simulink library "TripedLibrary"  (R2021a)
settings: Solver=VariableStepAuto  StartTime=0.0  StopTime=10.0  RelTol=1e-3
values from neighbouring files (symbols this model uses):
  s = 1/(2*r)    [Weg0.m]
undefined symbols (not defined in the file or in its folder): X, Y, Z
libraries: sm_lib x95, nesl_utility x42, $bdroot x14, robotlib x9, simulink x6, spsFirstOrderFilterLib x3, mspsensorlib x1
(part 5 of 5)

== matlab function TripedLibrary/Kinematic Utils/Simplified  Model Kinematics/Fwd Kin ==
  data: Jointstate input; leg_pos output; LegNumber input
function leg_pos = fcn(Jointstate, LegNumber)
waym = Weg0(eul2quat(Jointstate(1:3).','XYZ'));
wayLLm = AddLegLinear(waym,Jointstate(4));
legstate = getPosfromHomogenMatrix(wayLLm);
leg_pos = transformCoordinateSystem(legstate(1),legstate(2),legstate(3),LegNumber);
end




function [new_pos] = transformCoordinateSystem(oldx,oldy,oldz,legNr)
% this function translates the x,y,z coordinates from the CCS into
% coordinates from a cooridnate system, which is like the ccs but rotated
% ,such that its x axis points towards the leg. This makes the inverse
% kinematics for the leg 1 & 2 easier.

angle = -legNr * 120 * pi/180;

newCoord = [cos(angle), -sin(angle), 0, 0; sin(angle), cos(angle), 0, 0; 0, 0, 1, 0; 0, 0, 0, 1]* [oldx;oldy;oldz;1];
newx = newCoord(1);
newy = newCoord(2);
newz = newCoord(3);

new_pos=[newx;newy;newz];
end

function [Weg0Mat] = Weg0(quat)
a0=quat(1);
b0=quat(2);
c0=quat(3);
d0=quat(4);
A1 = homogenTranslationMat(0.265,0,0.014);
A2 = makeRotHomogen(quatRotM(a0,b0,c0,d0));
Weg0Mat = A1 * A2;
end



function [ALeg] = AddLegLinear(A,theta0)
% this functions adds transformations from the Point P; which is the
% Endpoint from Weg0,1,2; to the FKS at the LegLinear part.
%{
Inputs:
A: Transformationmatrix, which describes Transformation from HKS to P, Use
Weg0.m for that.
theta0: angle [radians] for joint at MKS00
%}

A1 = homogenTranslationMat(1.640, 0, -0.037); % transform P to P0 (center of LegLinear rotation)

theta0 = -1* theta0 * 0.07/(2*pi*1.5); % gear constraint: transfrom theta at MKS00 to theta around P0, gear ratio is 0.07/(2*pi*1.5) [circumferences of the gears MCS00 / LL]
startingvalue = -0 * pi/180;
theta0 = theta0 + startingvalue; %offset, depending on which position the Leg is for theta at MKS00 is 0
A2 = makeRotHomogen(quatRotM(cos(theta0/2),0,sin(theta0/2),0)); % rotate theta [radians] around y-axis of P0

A3 = homogenTranslationMat(-1.500,0,0); %transform from P0-joint to FKS

ALeg = A*A1*A2*A3;
end

function [res] = homogenTranslationMat(x,y,z)
    %this function forms a Translation about a vector x,y,z in a homogenous
    %transformation matrix res. 
    res = [1 0 0 x; 0 1 0 y; 0 0 1 z; 0 0 0 1];
end

function [res] = makeRotHomogen(R)
% this function fills a Rotationmatrix to make it a homogen transformation
% matrix
res = [R(1,1) R(1,2) R(1,3) 0; R(2,1) R(2,2) R(2,3) 0; R(3,1) R(3,2) R(3,3) 0; 0 0 0 1];
end

function [res] = quatRotM(a,b,c,d) %%Todo: use a,b,c,d as inputs
    % this function calculates the quaternion rotation matrix for given
    % vector (kx,ky,kz) and angle theta
    res = [1-2*(c^2+d^2) 2*(b*c-d*a) 2*(b*d + c*a); 2*(b*c + d*a) 1-2*(b^2+d^2) 2*(c*d - b*a); 2*(b*d-c*a) 2*(c*d+b*a) 1-2*(b^2+c^2) ];
end




function [pos] = getPosfromHomogenMatrix(A)
    % this function returns the Vector by which a homogenous
    % Transformationmatrix shifts a Point
    x = A(1,4);
    y = A(2,4);
    z = A(3,4);

    pos=[x,y,z];
end

== matlab function TripedLibrary/Kinematic Utils/Simplified  Model Kinematics/Inv Kin/Simplified_inverse_kinematics ==
  data: extend output; Rx output; Ry output; x input; y input; z input; LegAngle input; Rz output; data input; Residual output
function [extend,Rx,Ry,Rz,Residual]= fcn(x,y,z,LegAngle, data)



% easy adapt to legs 1 & 2: change base coordinate system from ccs, to
% rotated ccs.
[newx,newy,newz] = transformCoordinateSystem(x,y,z,LegAngle);

% calculate target Matrix from input cordinates
%reduced task space to x,y,z, ignore roll, pitch, yaw
[targetM] = convertCoordinatesToMatrix(newx,newy,newz);

%convert euer angles from data to quaternion
guess = convertDataToGuess(data);

[extend, a0,b0,c0,d0, Residual] = inverseKinematics(targetM,guess);
eulerXYZ = quat2eul([a0,b0,c0,d0],'XYZ');
Rx = eulerXYZ(1);
Ry = eulerXYZ(2);
Rz = eulerXYZ(3);

end

function [newx,newy,newz] = transformCoordinateSystem(oldx,oldy,oldz,legAngle)
% this function translates the x,y,z coordinates from the CCS into
% coordinates from a cooridnate system, which is like the ccs but rotated
% ,such that its x axis points towards the leg. This makes the inverse
% kinematics for the leg 1 & 2 easier.

angle = legAngle;

newCoord = [cos(angle), -sin(angle), 0, 0; sin(angle), cos(angle), 0, 0; 0, 0, 1, 0; 0, 0, 0, 1]* [oldx;oldy;oldz;1];
newx = newCoord(1);
newy = newCoord(2);
newz = newCoord(3);

end

function [transfM] = convertCoordinatesToMatrix(x,y,z)
transfM = homogenTranslationMat(x,y,z);
end

function [guess] = convertDataToGuess(data)
    qXYZ = eul2quat([data(1),data(2),data(3)],'XYZ');
    guess = [qXYZ,data(4)];    
end

function [theta0,a0,b0,c0,d0,fvalWay0] = inverseKinematics(A,guess)
% maps a homogene transformation matrix, which describes the desired position
% of the fcs relative to the ccs in taskspace to the joint space variables


options = optimoptions(@fmincon,'OptimalityTolerance',10^-10,'StepTolerance',10^-10,'display','off','Algorithm','sqp'); % some options for more precise solution


guessVals = guess;

clW0toTarget = @(guessVals)closingWay0toTarget(guessVals,A);
[OptVals,fvalWay0,~,~] = fmincon(clW0toTarget,guessVals,[],[],[],[],[],[],@constrainsWay0,options);

% get values from way0
a0 = OptVals(1);
b0 = OptVals(2);
c0 = OptVals(3);
d0 = OptVals(4);
theta0 = OptVals(5);

end


function [error] = closingWay0toTarget(GUESSEDVALS,MatA)
% this function returns the error between the desired fcs position and the
% fcs position given GUESSEDVALS as joint values

a0 = GUESSEDVALS(1);
b0 = GUESSEDVALS(2);
c0 = GUESSEDVALS(3);
d0 = GUESSEDVALS(4);
theta0 = GUESSEDVALS(5);

way0m = Weg0(a0,b0,c0,d0);
way0LLm = AddLegLinear(way0m,theta0);
[a,b,c,d, x,y,z] = getValuesfromHomogenMatrix(way0LLm);
[~,~,~,~, Ax,Ay,Az] = getValuesfromHomogenMatrix(MatA);


% give the system a desired yaw of the leg, since it is highly redundant
% this makes the solution more predictable

[~,desired_orientation]= cart2pol(Ax-0.265,Ay);
current_orientation = quat2eul([a0,b0,c0,d0]);


error = sum(([x,y,z] - [Ax,Ay,Az]).^2) + 1*(a^2+b^2+c^2+d^2 -1)^2+10*(desired_orientation-current_orientation(1))^2; % error of the transform to A. we want to minimze this
end


function [c,ceq]= constrainsWay0(x)
% make sure that solver fmincon considers that the quaternion a0,b0,c0,d0
% needs to be normalized.
%input: x = [a0,b0,c0,d0,theta0].
c = []; % condition for ... <= 0
ceq = x(1)^2+x(2)^2+x(3)^2+x(4)^2 - 1; % condition for ||quat0|| == 1    
end

function [Weg0Mat] = Weg0(a0,b0,c0,d0)
A1 = homogenTranslationMat(0.265,0,0.014);
A2 = makeRotHomogen(quatRotM(a0,b0,c0,d0));
Weg0Mat = A1 * A2;
end

function [ALeg] = AddLegLinear(A,theta0)
% this functions adds transformations from the Point P; which is the
% Endpoint from Weg0,1,2; to the FKS at the LegLinear part.
%{
Inputs:
A: Transformationmatrix, which describes Transformation from HKS to P, Use
Weg0.m for that.
theta0: angle [radians] for joint at MKS00
%}

A1 = homogenTranslationMat(1.640, 0, -0.037); 

theta0 = -1* theta0 * 0.07/(2*pi*1.5); % gear constraint between motor and curved leg
startingvalue = -0 * pi/180;
theta0 = theta0 + startingvalue;
A2 = makeRotHomogen(quatRotM(cos(theta0/2),0,sin(theta0/2),0)); 
A3 = homogenTranslationMat(-1.500,0,0);

ALeg = A*A1*A2*A3;
end

function [res] = homogenTranslationMat(x,y,z)
    %this function forms a Translation about a vector x,y,z in a homogenous
    %transformation matrix res. 
    res = [1 0 0 x; 0 1 0 y; 0 0 1 z; 0 0 0 1];
end

function [res] = makeRotHomogen(R)
% this function fills a Rotationmatrix to make it a homogen transformation
% matrix
res = [R(1,1) R(1,2) R(1,3) 0; R(2,1) R(2,2) R(2,3) 0; R(3,1) R(3,2) R(3,3) 0; 0 0 0 1];
end

function [res] = quatRotM(a,b,c,d) %%Todo: use a,b,c,d as inputs
    res = [1-2*(c^2+d^2) 2*(b*c-d*a) 2*(b*d + c*a); 2*(b*c + d*a) 1-2*(b^2+d^2) 2*(c*d - b*a); 2*(b*d-c*a) 2*(c*d+b*a) 1-2*(b^2+c^2) ];
end

function [a,b,c,d, x,y,z] = getValuesfromHomogenMatrix(A)
    % this function returns the Vector by which a homogenous
    % Transformationmatrix shifts a Point
    x = A(1,4);
    y = A(2,4);
    z = A(3,4);

    %as well as the Values of the Quaternion describing the rotation
    R = A(1:3,1:3); % get Rot mat from homogen Mat
    quat = rotm2quat(R);
    a = quat(1);
    b = quat(2);
    c = quat(3);
    d = quat(4); 
end

== matlab function TripedLibrary/Kinematic Utils/fullbody kinematics ==
  data: foot0 input; res output; foot1 input; foot2 input; roll input; pitch input; yaw input; height input
function res  = fcn(foot0,foot1,foot2,roll,pitch,yaw,height)
floor_ccs_trafo=transform_to_floor(roll,pitch,yaw,height);

ccs_foot0=floor_ccs_trafo*makehomogenous(foot0);
ccs_foot1=floor_ccs_trafo*makehomogenous(foot1);
ccs_foot2=floor_ccs_trafo*makehomogenous(foot2);
res=[ccs_foot0(1:3);ccs_foot1(1:3);ccs_foot2(1:3)];
end


function [transfM] = transform_to_floor(roll,pitch,yaw,height)
%first translate frame by [x,y,z]
transfM1 = homogenTranslationMat(0,0,-height);
%then rotate using the roll-pitch-yaw convention
transfM2 = makeRotHomogen(eul2rotm([-roll,-pitch,-yaw],'XYZ'));
transfM = transfM1 * transfM2;
end

function [res] = makehomogenous(vector)
    res = [vector(1);vector(2);vector(3);1];
end

function [res] = homogenTranslationMat(x,y,z)
    %this function forms a Translation about a vector x,y,z in a homogenous
    %transformation matrix res. 
    res = [1 0 0 x; 0 1 0 y; 0 0 1 z; 0 0 0 1];
end

function [res] = makeRotHomogen(R)
% this function fills a Rotationmatrix to make it a homogen transformation
% matrix
res = [R(1,1) R(1,2) R(1,3) 0; R(2,1) R(2,2) R(2,3) 0; R(3,1) R(3,2) R(3,3) 0; 0 0 0 1];
end

== matlab function TripedLibrary/Simplified Model/TriPed/Forward Kinematics/MATLAB Function ==
  data: Jointstate input; leg_pos output; LegNumber input
function leg_pos = fcn(Jointstate, LegNumber)
waym = Weg0(eul2quat(Jointstate(1:3).','XYZ'));
wayLLm = AddLegLinear(waym,Jointstate(4));
legstate = getPosfromHomogenMatrix(wayLLm);
leg_pos = transformCoordinateSystem(legstate(1),legstate(2),legstate(3),LegNumber);
end




function [new_pos] = transformCoordinateSystem(oldx,oldy,oldz,legNr)
% this function translates the x,y,z coordinates from the CCS into
% coordinates from a cooridnate system, which is like the ccs but rotated
% ,such that its x axis points towards the leg. This makes the inverse
% kinematics for the leg 1 & 2 easier.

angle = -legNr * 120 * pi/180;

newCoord = [cos(angle), -sin(angle), 0, 0; sin(angle), cos(angle), 0, 0; 0, 0, 1, 0; 0, 0, 0, 1]* [oldx;oldy;oldz;1];
newx = newCoord(1);
newy = newCoord(2);
newz = newCoord(3);

new_pos=[newx;newy;newz];
end

function [Weg0Mat] = Weg0(quat)
a0=quat(1);
b0=quat(2);
c0=quat(3);
d0=quat(4);
A1 = homogenTranslationMat(0.265,0,0.014);
A2 = makeRotHomogen(quatRotM(a0,b0,c0,d0));
Weg0Mat = A1 * A2;
end



function [ALeg] = AddLegLinear(A,theta0)
% this functions adds transformations from the Point P; which is the
% Endpoint from Weg0,1,2; to the FKS at the LegLinear part.
%{
Inputs:
A: Transformationmatrix, which describes Transformation from HKS to P, Use
Weg0.m for that.
theta0: angle [radians] for joint at MKS00
%}

A1 = homogenTranslationMat(1.640, 0, -0.037); % transform P to P0 (center of LegLinear rotation)

theta0 = -1* theta0 * 0.07/(2*pi*1.5); % gear constraint: transfrom theta at MKS00 to theta around P0, gear ratio is 0.07/(2*pi*1.5) [circumferences of the gears MCS00 / LL]
startingvalue = -0 * pi/180;
theta0 = theta0 + startingvalue; %offset, depending on which position the Leg is for theta at MKS00 is 0
A2 = makeRotHomogen(quatRotM(cos(theta0/2),0,sin(theta0/2),0)); % rotate theta [radians] around y-axis of P0

A3 = homogenTranslationMat(-1.500,0,0); %transform from P0-joint to FKS

ALeg = A*A1*A2*A3;
end

function [res] = homogenTranslationMat(x,y,z)
    %this function forms a Translation about a vector x,y,z in a homogenous
    %transformation matrix res. 
    res = [1 0 0 x; 0 1 0 y; 0 0 1 z; 0 0 0 1];
end

function [res] = makeRotHomogen(R)
% this function fills a Rotationmatrix to make it a homogen transformation
% matrix
res = [R(1,1) R(1,2) R(1,3) 0; R(2,1) R(2,2) R(2,3) 0; R(3,1) R(3,2) R(3,3) 0; 0 0 0 1];
end

function [res] = quatRotM(a,b,c,d) %%Todo: use a,b,c,d as inputs
    % this function calculates the quaternion rotation matrix for given
    % vector (kx,ky,kz) and angle theta
    res = [1-2*(c^2+d^2) 2*(b*c-d*a) 2*(b*d + c*a); 2*(b*c + d*a) 1-2*(b^2+d^2) 2*(c*d - b*a); 2*(b*d-c*a) 2*(c*d+b*a) 1-2*(b^2+c^2) ];
end




function [pos] = getPosfromHomogenMatrix(A)
    % this function returns the Vector by which a homogenous
    % Transformationmatrix shifts a Point
    x = A(1,4);
    y = A(2,4);
    z = A(3,4);

    pos=[x,y,z];
end

== matlab function TripedLibrary/Full Model/ROS/Publisher_leg_0/Sensor_Publisher/mergeValuesIntoRosMsg_test ==
  data: blankMessage input Bus: SL_Bus_triped_sensor_msgs_JointState; position input; msg output Bus: SL_Bus_triped_sensor_msgs_JointState
function msg = assignNestedArrayMessages(blankMessage,position)
%#codegen

% To set datatype of MSG output:
%  1. Create buses for this model: robotics.ros.createSimulinkBus(gcs)
%  1. Click "Edit Data" in  Toolstrip to open "Ports and Data Manager"
%  2. Select MSG and set datatype to "Bus: SL_Bus_<modelname>_<messageType>"
% See: 
% http://www.mathworks.com/help/simulink/ug/create-structures-in-matlab-function-blocks.html

% blankMessage (geometry_msgs/PoseArray) consists of
%          Header: [1x1 Header]
%           Poses: variable-length array of geometry_msgs/Pose
%   Poses_SL_Info: struct with fields CurrentLength, ReceivedLength
%
% Poses is an array of "geometry_msgs/Pose", which consists of
%        Position: [1x1 Point]
%     Orientation: [1x1 Quaternion]
%
% Position is "geometry_msgs/Point", which consists of
%               X: 0
%               Y: 0
%               Z: 0
%
% Orientation is "geometry_msgs/Quaternion", which consists of
%               X: 0
%               Y: 0
%               Z: 0
%               W: 0

% Set the Poses array to have size 2, and modify the first two Pose
% elements

%blankMessage.Poses_SL_Info.CurrentLength = uint32(2);
%blankMessage.Poses(1).Position.X = x;
%blankMessage.Poses(1).Position.Y = y;
%blankMessage.Poses(2).Orientation.Z = z;

blankMessage.Position_SL_Info.CurrentLength = uint32(1);
%blankMessage.Velocity_SL_Info.CurrentLength = uint32(2);
%blankMessage.Effort_SL_Info.CurrentLength = uint32(2);
blankMessage.Position(1) = position;
%blankMessage.Velocity(2) = velocity;
%blankMessage.Position(2) = effort;

msg = blankMessage;

== matlab function TripedLibrary/Simplified Model/TriPed/Forward Kinematics/MATLAB Function1 ==
  data: Jointstate input; leg_pos output; LegNumber input
function leg_pos = fcn(Jointstate, LegNumber)
waym = Weg0(eul2quat(Jointstate(1:3).','XYZ'));
wayLLm = AddLegLinear(waym,Jointstate(4));
legstate = getPosfromHomogenMatrix(wayLLm);
leg_pos = transformCoordinateSystem(legstate(1),legstate(2),legstate(3),LegNumber);
end




function [new_pos] = transformCoordinateSystem(oldx,oldy,oldz,legNr)
% this function translates the x,y,z coordinates from the CCS into
% coordinates from a cooridnate system, which is like the ccs but rotated
% ,such that its x axis points towards the leg. This makes the inverse
% kinematics for the leg 1 & 2 easier.

angle = -legNr * 120 * pi/180;

newCoord = [cos(angle), -sin(angle), 0, 0; sin(angle), cos(angle), 0, 0; 0, 0, 1, 0; 0, 0, 0, 1]* [oldx;oldy;oldz;1];
newx = newCoord(1);
newy = newCoord(2);
newz = newCoord(3);

new_pos=[newx;newy;newz];
end

function [Weg0Mat] = Weg0(quat)
a0=quat(1);
b0=quat(2);
c0=quat(3);
d0=quat(4);
A1 = homogenTranslationMat(0.265,0,0.014);
A2 = makeRotHomogen(quatRotM(a0,b0,c0,d0));
Weg0Mat = A1 * A2;
end



function [ALeg] = AddLegLinear(A,theta0)
% this functions adds transformations from the Point P; which is the
% Endpoint from Weg0,1,2; to the FKS at the LegLinear part.
%{
Inputs:
A: Transformationmatrix, which describes Transformation from HKS to P, Use
Weg0.m for that.
theta0: angle [radians] for joint at MKS00
%}

A1 = homogenTranslationMat(1.640, 0, -0.037); % transform P to P0 (center of LegLinear rotation)

theta0 = -1* theta0 * 0.07/(2*pi*1.5); % gear constraint: transfrom theta at MKS00 to theta around P0, gear ratio is 0.07/(2*pi*1.5) [circumferences of the gears MCS00 / LL]
startingvalue = -0 * pi/180;
theta0 = theta0 + startingvalue; %offset, depending on which position the Leg is for theta at MKS00 is 0
A2 = makeRotHomogen(quatRotM(cos(theta0/2),0,sin(theta0/2),0)); % rotate theta [radians] around y-axis of P0

A3 = homogenTranslationMat(-1.500,0,0); %transform from P0-joint to FKS

ALeg = A*A1*A2*A3;
end

function [res] = homogenTranslationMat(x,y,z)
    %this function forms a Translation about a vector x,y,z in a homogenous
    %transformation matrix res. 
    res = [1 0 0 x; 0 1 0 y; 0 0 1 z; 0 0 0 1];
end

function [res] = makeRotHomogen(R)
% this function fills a Rotationmatrix to make it a homogen transformation
% matrix
res = [R(1,1) R(1,2) R(1,3) 0; R(2,1) R(2,2) R(2,3) 0; R(3,1) R(3,2) R(3,3) 0; 0 0 0 1];
end

function [res] = quatRotM(a,b,c,d) %%Todo: use a,b,c,d as inputs
    % this function calculates the quaternion rotation matrix for given
    % vector (kx,ky,kz) and angle theta
    res = [1-2*(c^2+d^2) 2*(b*c-d*a) 2*(b*d + c*a); 2*(b*c + d*a) 1-2*(b^2+d^2) 2*(c*d - b*a); 2*(b*d-c*a) 2*(c*d+b*a) 1-2*(b^2+c^2) ];
end




function [pos] = getPosfromHomogenMatrix(A)
    % this function returns the Vector by which a homogenous
    % Transformationmatrix shifts a Point
    x = A(1,4);
    y = A(2,4);
    z = A(3,4);

    pos=[x,y,z];
end

== matlab function TripedLibrary/Simplified Model/TriPed/Forward Kinematics/MATLAB Function2 ==
  data: Jointstate input; leg_pos output; LegNumber input
function leg_pos = fcn(Jointstate, LegNumber)
waym = Weg0(eul2quat(Jointstate(1:3).','XYZ'));
wayLLm = AddLegLinear(waym,Jointstate(4));
legstate = getPosfromHomogenMatrix(wayLLm);
leg_pos = transformCoordinateSystem(legstate(1),legstate(2),legstate(3),LegNumber);
end




function [new_pos] = transformCoordinateSystem(oldx,oldy,oldz,legNr)
% this function translates the x,y,z coordinates from the CCS into
% coordinates from a cooridnate system, which is like the ccs but rotated
% ,such that its x axis points towards the leg. This makes the inverse
% kinematics for the leg 1 & 2 easier.

angle = -legNr * 120 * pi/180;

newCoord = [cos(angle), -sin(angle), 0, 0; sin(angle), cos(angle), 0, 0; 0, 0, 1, 0; 0, 0, 0, 1]* [oldx;oldy;oldz;1];
newx = newCoord(1);
newy = newCoord(2);
newz = newCoord(3);

new_pos=[newx;newy;newz];
end

function [Weg0Mat] = Weg0(quat)
a0=quat(1);
b0=quat(2);
c0=quat(3);
d0=quat(4);
A1 = homogenTranslationMat(0.265,0,0.014);
A2 = makeRotHomogen(quatRotM(a0,b0,c0,d0));
Weg0Mat = A1 * A2;
end



function [ALeg] = AddLegLinear(A,theta0)
% this functions adds transformations from the Point P; which is the
% Endpoint from Weg0,1,2; to the FKS at the LegLinear part.
%{
Inputs:
A: Transformationmatrix, which describes Transformation from HKS to P, Use
Weg0.m for that.
theta0: angle [radians] for joint at MKS00
%}

A1 = homogenTranslationMat(1.640, 0, -0.037); % transform P to P0 (center of LegLinear rotation)

theta0 = -1* theta0 * 0.07/(2*pi*1.5); % gear constraint: transfrom theta at MKS00 to theta around P0, gear ratio is 0.07/(2*pi*1.5) [circumferences of the gears MCS00 / LL]
startingvalue = -0 * pi/180;
theta0 = theta0 + startingvalue; %offset, depending on which position the Leg is for theta at MKS00 is 0
A2 = makeRotHomogen(quatRotM(cos(theta0/2),0,sin(theta0/2),0)); % rotate theta [radians] around y-axis of P0

A3 = homogenTranslationMat(-1.500,0,0); %transform from P0-joint to FKS

ALeg = A*A1*A2*A3;
end

function [res] = homogenTranslationMat(x,y,z)
    %this function forms a Translation about a vector x,y,z in a homogenous
    %transformation matrix res. 
    res = [1 0 0 x; 0 1 0 y; 0 0 1 z; 0 0 0 1];
end

function [res] = makeRotHomogen(R)
% this function fills a Rotationmatrix to make it a homogen transformation
% matrix
res = [R(1,1) R(1,2) R(1,3) 0; R(2,1) R(2,2) R(2,3) 0; R(3,1) R(3,2) R(3,3) 0; 0 0 0 1];
end

function [res] = quatRotM(a,b,c,d) %%Todo: use a,b,c,d as inputs
    % this function calculates the quaternion rotation matrix for given
    % vector (kx,ky,kz) and angle theta
    res = [1-2*(c^2+d^2) 2*(b*c-d*a) 2*(b*d + c*a); 2*(b*c + d*a) 1-2*(b^2+d^2) 2*(c*d - b*a); 2*(b*d-c*a) 2*(c*d+b*a) 1-2*(b^2+c^2) ];
end




function [pos] = getPosfromHomogenMatrix(A)
    % this function returns the Vector by which a homogenous
    % Transformationmatrix shifts a Point
    x = A(1,4);
    y = A(2,4);
    z = A(3,4);

    pos=[x,y,z];
end

== matlab function TripedLibrary/Full Model/ROS/Publisher_leg_0/Sensor_Publisher1/mergeValuesIntoRosMsg_test ==
  data: blankMessage input Bus: SL_Bus_triped_sensor_msgs_JointState; position input; msg output Bus: SL_Bus_triped_sensor_msgs_JointState
function msg = assignNestedArrayMessages(blankMessage,position)
%#codegen

% To set datatype of MSG output:
%  1. Create buses for this model: robotics.ros.createSimulinkBus(gcs)
%  1. Click "Edit Data" in  Toolstrip to open "Ports and Data Manager"
%  2. Select MSG and set datatype to "Bus: SL_Bus_<modelname>_<messageType>"
% See: 
% http://www.mathworks.com/help/simulink/ug/create-structures-in-matlab-function-blocks.html

% blankMessage (geometry_msgs/PoseArray) consists of
%          Header: [1x1 Header]
%           Poses: variable-length array of geometry_msgs/Pose
%   Poses_SL_Info: struct with fields CurrentLength, ReceivedLength
%
% Poses is an array of "geometry_msgs/Pose", which consists of
%        Position: [1x1 Point]
%     Orientation: [1x1 Quaternion]
%
% Position is "geometry_msgs/Point", which consists of
%               X: 0
%               Y: 0
%               Z: 0
%
% Orientation is "geometry_msgs/Quaternion", which consists of
%               X: 0
%               Y: 0
%               Z: 0
%               W: 0

% Set the Poses array to have size 2, and modify the first two Pose
% elements

%blankMessage.Poses_SL_Info.CurrentLength = uint32(2);
%blankMessage.Poses(1).Position.X = x;
%blankMessage.Poses(1).Position.Y = y;
%blankMessage.Poses(2).Orientation.Z = z;

blankMessage.Position_SL_Info.CurrentLength = uint32(1);
%blankMessage.Velocity_SL_Info.CurrentLength = uint32(2);
%blankMessage.Effort_SL_Info.CurrentLength = uint32(2);
blankMessage.Position(1) = position;
%blankMessage.Velocity(2) = velocity;
%blankMessage.Position(2) = effort;

msg = blankMessage;

== matlab function TripedLibrary/Full Model/ROS/Publisher_leg_0/Sensor_Publisher2/mergeValuesIntoRosMsg_test ==
  data: blankMessage input Bus: SL_Bus_triped_sensor_msgs_JointState; position input; msg output Bus: SL_Bus_triped_sensor_msgs_JointState
function msg = assignNestedArrayMessages(blankMessage,position)
%#codegen

% To set datatype of MSG output:
%  1. Create buses for this model: robotics.ros.createSimulinkBus(gcs)
%  1. Click "Edit Data" in  Toolstrip to open "Ports and Data Manager"
%  2. Select MSG and set datatype to "Bus: SL_Bus_<modelname>_<messageType>"
% See: 
% http://www.mathworks.com/help/simulink/ug/create-structures-in-matlab-function-blocks.html

% blankMessage (geometry_msgs/PoseArray) consists of
%          Header: [1x1 Header]
%           Poses: variable-length array of geometry_msgs/Pose
%   Poses_SL_Info: struct with fields CurrentLength, ReceivedLength
%
% Poses is an array of "geometry_msgs/Pose", which consists of
%        Position: [1x1 Point]
%     Orientation: [1x1 Quaternion]
%
% Position is "geometry_msgs/Point", which consists of
%               X: 0
%               Y: 0
%               Z: 0
%
% Orientation is "geometry_msgs/Quaternion", which consists of
%               X: 0
%               Y: 0
%               Z: 0
%               W: 0

% Set the Poses array to have size 2, and modify the first two Pose
% elements

%blankMessage.Poses_SL_Info.CurrentLength = uint32(2);
%blankMessage.Poses(1).Position.X = x;
%blankMessage.Poses(1).Position.Y = y;
%blankMessage.Poses(2).Orientation.Z = z;

blankMessage.Position_SL_Info.CurrentLength = uint32(1);
%blankMessage.Velocity_SL_Info.CurrentLength = uint32(2);
%blankMessage.Effort_SL_Info.CurrentLength = uint32(2);
blankMessage.Position(1) = position;
%blankMessage.Velocity(2) = velocity;
%blankMessage.Position(2) = effort;

msg = blankMessage;

== matlab function TripedLibrary/Examples/Full Body orientation and height control/fullbody kinematics ==
  data: foot0 input; res output; foot1 input; foot2 input; roll input; pitch input; yaw input; height input
function res  = fcn(foot0,foot1,foot2,roll,pitch,yaw,height)
floor_ccs_trafo=transform_to_floor(roll,pitch,yaw,height);

ccs_foot0=floor_ccs_trafo*makehomogenous(foot0);
ccs_foot1=floor_ccs_trafo*makehomogenous(foot1);
ccs_foot2=floor_ccs_trafo*makehomogenous(foot2);
res=[ccs_foot0(1:3);ccs_foot1(1:3);ccs_foot2(1:3)];
end


function [transfM] = transform_to_floor(roll,pitch,yaw,height)
%first translate frame by [x,y,z]
transfM1 = homogenTranslationMat(0,0,-height);
%then rotate using the roll-pitch-yaw convention
transfM2 = makeRotHomogen(eul2rotm([-roll,-pitch,-yaw],'XYZ'));
transfM = transfM1 * transfM2;
end

function [res] = makehomogenous(vector)
    res = [vector(1);vector(2);vector(3);1];
end

function [res] = homogenTranslationMat(x,y,z)
    %this function forms a Translation about a vector x,y,z in a homogenous
    %transformation matrix res. 
    res = [1 0 0 x; 0 1 0 y; 0 0 1 z; 0 0 0 1];
end

function [res] = makeRotHomogen(R)
% this function fills a Rotationmatrix to make it a homogen transformation
% matrix
res = [R(1,1) R(1,2) R(1,3) 0; R(2,1) R(2,2) R(2,3) 0; R(3,1) R(3,2) R(3,3) 0; 0 0 0 1];
end

== matlab function TripedLibrary/Examples/Spider Walking/Gait Generator ==
  data: foot_0 output; foot_1 output; foot_2 output; current_foot_pos input; angle output; angle input; walking_dir input
function [foot_0,foot_1,foot_2,angle] = fcn(current_foot_pos,angle,walking_dir)
    timestep  = 0.01;
    duration  = 0.5;
    height    = 0.08;
    dt        = timestep/duration;
    increment = 3/3*pi;
    swing_rad = 0.10;
    velocity  = 0.2;

    initial_pos_0 = [0.4    ; 0       ; -0.6]*1.1;
    initial_pos_1 = [-0.2025; -0.35074; -0.6]*1.1;
    initial_pos_2 = [-0.2025;  0.35074; -0.6]*1.1;
    
    init_angle_0  = mod(2*pi/360* 0   + 0*pi/2,2*pi);
    init_angle_1  = mod(2*pi/360* 240 + 0*pi/2,2*pi); %angle convention other direction for some reason
    init_angle_2  = mod(2*pi/360* 120 + 0*pi/2,2*pi);
    
    
    rel_step_angle= 60;
    final_angle_0 = mod(init_angle_0+2*pi/360*rel_step_angle,2*pi);
    final_angle_1 = mod(init_angle_1+2*pi/360*rel_step_angle,2*pi);
    final_angle_2 = mod(init_angle_2+2*pi/360*rel_step_angle,2*pi);
    
    angle       = angle+increment*timestep;
    angle_setup = walking_dir/360*2*pi;
    if angle >= 3*pi
        foot_0 = initial_pos_0 + swing_rad * [cos(angle_setup);sin(angle_setup);0];
        foot_1 = initial_pos_1 + swing_rad * [cos(angle_setup);sin(angle_setup);0];
        foot_2 = initial_pos_2 + swing_rad * [cos(angle_setup);sin(angle_setup);0];
        
        if angle >=4*pi
            angle = angle_setup;
        end
    else
        angle = mod(angle,2*pi);

        [foot_0] = single_leg_state(current_foot_pos(1:3),initial_pos_0,height,angle,swing_rad,final_angle_0,velocity,init_angle_0,walking_dir);
        [foot_1] = single_leg_state(current_foot_pos(4:6),initial_pos_1,height,angle,swing_rad,final_angle_1,velocity,init_angle_1,walking_dir);  
        [foot_2] = single_leg_state(current_foot_pos(7:9),initial_pos_2,height,angle,swing_rad,final_angle_2,velocity,init_angle_2,walking_dir);
    end
end


function [foot]=single_leg_state(foot_pos,initial_pos,height,angle,swing_rad,final_angle,velocity,init_angle,walking_dir)
    final_pos    = initial_pos+swing_rad*[cos(final_angle);sin(final_angle);0];
    stepping_pos = initial_pos+swing_rad*[cos(init_angle) ;sin(init_angle) ;0]-rotz(walking_dir)*[1;0;0]*(angle-final_angle+2*pi)/(2*pi)*velocity;
    
    if (angle >=init_angle) &&(angle <=final_angle)
        s = (angle-init_angle)/(final_angle-init_angle); %state jump here might make the system jump out of s if final angle is after zero crossing
        foot = targeted_step(s,height,stepping_pos,final_pos);
    else
        if angle-final_angle >=0
            move_memory=angle-final_angle;
        else
            move_memory=angle-final_angle+2*pi;
        end
        foot = initial_pos+swing_rad*[cos(angle);sin(angle);0]-rotz(walking_dir)*[1;0;0]*move_memory/(2*pi)*velocity; %TODO should be full roll pitch yaw control
    end
end

function foot_position=targeted_step(s,height,start,stop)
    relative_pos  = stop-start;
    [rot,len]   = cart2pol(relative_pos(1),relative_pos(2));
    foot_position = rotz(rot/(2*pi)*360)*step(s,len,height)+start;
end

function foot_position=step(s,length,height)
a = 0;%16*height;
b = 0;%0;
c = -4*height;%-8*height;
d = 0;%height;
e = height;%1.5*height;

z = a*(s-0.5)^4 + b*(s-0.5)^3 + c*(s-0.5)^2 + d*(s-0.5) + e;
x = 0.5* length*(1+(sign(s-0.5)*sqrt(1-z^2/height^2)));
y = 0; %can be calculated from x using rotation matrix for different ori.

foot_position = [x; y; z];
end
